simulink model "pompa"  (R2022b)
settings: Solver=VariableStepAuto  StartTime=0.0  StopTime=10.0  RelTol=1e-3
values from neighbouring files (symbols this model uses):
  k11 = k2^2 + 4*(k - k3)*k1    (= 0.08909684)    [date_indrumator.m]    (also in proiect.m = 0.08885985)
  k12 = 8*(k-k3)    (= 0.2848)    [date_indrumator.m]    (also in proiect.m)
  k13 = 2*(k-k3)    (= 0.0712)    [date_indrumator.m]    (also in proiect.m)
  k2 = -0.015    [date_indrumator.m]    (also in proiect.m = -0.0015)
settings Model: Creator=Ruxandra  LastModifiedBy=Ruxandra

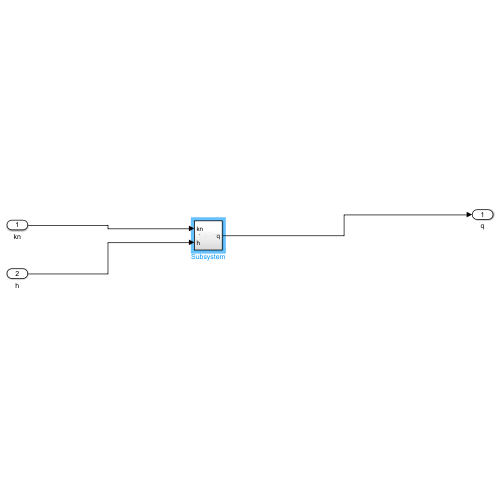
[thumbnail: Simulink's stored preview of the top-level diagram]
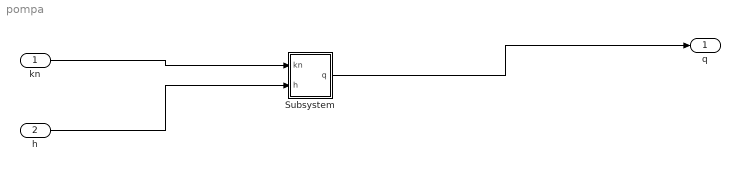
== system pompa ==
  kn : Inport
  h : Inport  Port=2
  Subsystem : Subsystem
  q : Outport
  wires:
  kn/1 -> Subsystem/1(kn)
  h/1 -> Subsystem/2(h)
  Subsystem/1(q) -> q/1

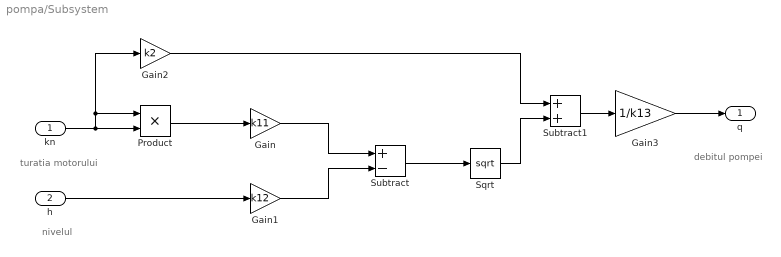
== system pompa/Subsystem ==
  note: debitul pompei
  note: nivelul
  note: turatia motorului
  kn : Inport
  h : Inport  Port=2
  Gain : Gain  Gain=k11
  Gain1 : Gain  Gain=k12
  Gain2 : Gain  Gain=k2
  Gain3 : Gain  Gain=1/k13
  Product : Product
  Sqrt : Sqrt
  Subtract : Sum  Inputs=+-
  Subtract1 : Sum
  q : Outport
  wires:
  Sqrt/1 -> Subtract1/2
  Gain1/1 -> Subtract/2
  h/1 -> Gain1/1
  Gain2/1 -> Subtract1/1
  kn/1 -> Product/1, Gain2/1, Product/2
  Subtract/1 -> Sqrt/1
  Subtract1/1 -> Gain3/1
  Gain/1 -> Subtract/1
  Gain3/1 -> q/1
  Product/1 -> Gain/1
